simulink model "openloop_motor_with_sources_2020a"  (R2022a)
settings: Solver=VariableStepAuto  StartTime=0.0  StopTime=2  MaxStep=1e-6  MinStep=1e-12  RelTol=1e-3
values from neighbouring files (symbols this model uses):
  J = 0.02    [parameter.mat]
  Llr = 0.01033    [parameter.mat]
  Lls = 0.01033    [parameter.mat]
  Lm = 0.3197    [parameter.mat]
  Lr = 0.33003    [parameter.mat]
  Ls = 0.33003    [parameter.mat]
  np = 2    [parameter.mat]
  Rr = 2.178    [parameter.mat]
  Rs = 2.804    [parameter.mat]
  Tr = 0.15152892562    [parameter.mat]
undefined symbols (not defined in the file or in its folder): f, theta
libraries: spsACVoltageSourceLib x3, spsVoltageMeasurementLib x3, spsGroundLib x2, spsAsynchronousMachineSIUnitsLib x1, spspowerguiLib x1
settings Model: Creator=EVA  LastModifiedBy=EVA
settings SolverCC: AlgebraicLoopSolver=TrustRegion

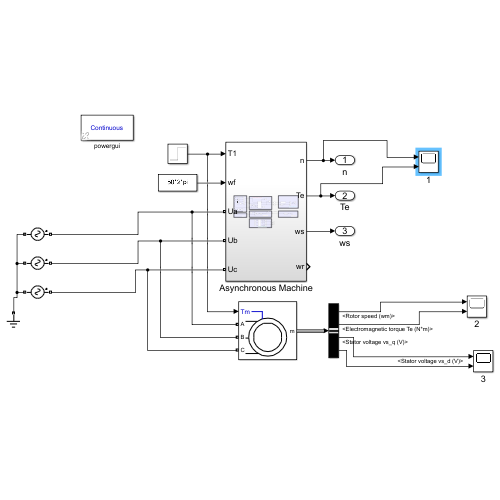
[thumbnail: Simulink's stored preview of the top-level diagram]
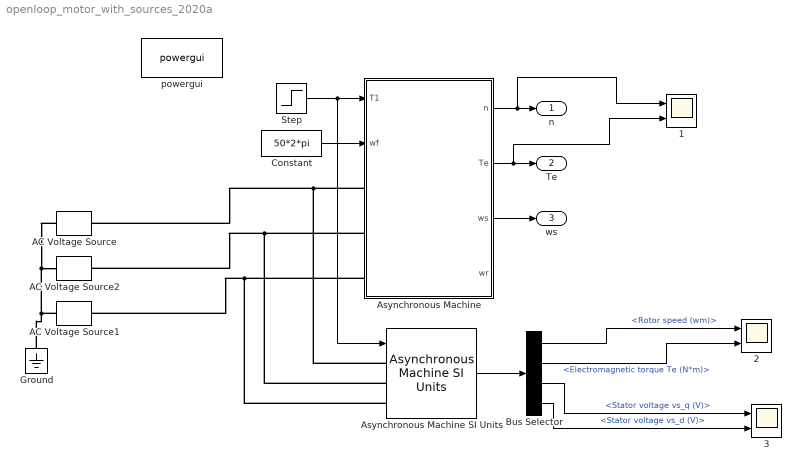
== system openloop_motor_with_sources_2020a ==
  1 : Scope  NumInputPorts=2
  2 : Scope  NumInputPorts=2
  3 : Scope  NumInputPorts=2
  AC Voltage Source : spsACVoltageSourceLib/AC Voltage Source  Amplitude=380  Phase=theta  Frequency=50  SampleTime=0  Measurements=None  BusType=swing  Pref=10e3  Qref=0  Qmin=-inf  Qmax=+inf
  AC Voltage Source1 : spsACVoltageSourceLib/AC Voltage Source  Amplitude=380  Phase=-240+theta  Frequency=50  SampleTime=0  Measurements=None  BusType=swing  Pref=10e3  Qref=0  Qmin=-inf  Qmax=+inf
  AC Voltage Source2 : spsACVoltageSourceLib/AC Voltage Source  Amplitude=380  Phase=-120+theta  Frequency=50  SampleTime=0  Measurements=None  BusType=swing  Pref=10e3  Qref=0  Qmin=-inf  Qmax=+inf
  Asynchronous Machine : Subsystem
  Asynchronous Machine SI Units : spsAsynchronousMachineSIUnitsLib/Asynchronous Machine SI Units  RotorType=Squirrel-cage  PresetModel=No  MechanicalLoad=Torque Tm  ShowDetailedParameters=on  ReferenceFrame=Rotor  Units=SI  MeasurementBus=off  NominalParameters=[1.845e+03 268 f]  VoltageRatio=1  Stator=[Rs Lls]  Rotor=[Rr Llr]  Cage1=[0.4155 0.002066]  Cage2=[0.4168 0.0003495]  Lm=Lm  Mechanical=[J 0.0 np]  PolePairs=2  InitialConditions=[1 0 0 0 0 0 0 0]  SimulateSaturation=off  Saturation=[14.03593122, 27.81365428, 53.79336849, 72.68890987, 97.98006896, 148.6815601, 215.7428561, 302.9841135, 428.7778367 ; 230, 322, 414, 460, 506, 552, 598, 644, 690]  LoadFlowParameters=1492000  TsPowergui=0  TsBlock=-1  IterativeModel=Trapezoidal non iterative  IterativeDiscreteModel=Trapezoidal non iterative  Pmec=0
  Bus Selector : BusSelector  OutputSignals=Mechanical.Rotor speed (wm),Mechanical.Electromagnetic torque Te (N*m),Stator measurements.Stator voltage vs_q (V),Stator measurements.Stator voltage vs_d (V)
  Constant : Constant  Value=50*2*pi
  Ground : spsGroundLib/Ground  LConnTagsString=a
  Step : Step  After=5  SampleTime=0
  powergui : spspowerguiLib/powergui  Priority=1  SimulationMode=Continuous  SampleTime=1e-7  frequency=60  Iterations=50  frequencyindice=50  Pbase=100e6  ErrMax=1e-4  UnitsV=kV  UnitsW=MW  buscounter=0  FunctionMessages=off  echomessages=off  EnableUseOfTLC=off  CurrentSourceSwitches=off  DisableSnubberDevices=off  DisableRonSwitches=off  DisableVfSwitches=off  DisplayEquations=off  AutomaticDiscreteSolvers=off  SolverType=Tustin/Backward Euler (TBE)  Interpol=off  ExternalGateDelay=off  methode=off  Ts=100  x0status=blocks  SPID=on  SwTol=0  HookPort=off  NonlinearTolerance=1e-4  nMaxIteration=100  ContinueOnMaxIteration=off  RestoreLinks=warning  ResistiveCurrentMeasurement=off  Frange=[0:2:500]  Ylog=off  Xlog=on  ShowGrid=off  save=off  variable=ZData  structure=0  ZoomFFT=off  StartTime=0.0  cycles=1  DisplayStyle=1  fundamental=60  FreqAxis=off  MaxFrequency=1000  frequencyindicesteady=1  RmsSteady=1  display=off
  n : Outport
  Te : Outport  Port=2
  ws : Outport  Port=3
  wires:
  Asynchronous Machine/1(n) -> 1/1, n/1
  Constant/1 -> Asynchronous Machine/2(wf)
  Asynchronous Machine/2(Te) -> 1/2, Te/1
  Step/1 -> Asynchronous Machine SI Units/1, Asynchronous Machine/1(T1)
  Asynchronous Machine/3(ws) -> ws/1
  Asynchronous Machine SI Units/1 -> Bus Selector/1
  Bus Selector/1 -> 2/1  "<Rotor speed (wm)>"
  Bus Selector/2 -> 2/2  "<Electromagnetic torque Te (N*m)>"
  Bus Selector/3 -> 3/1  "<Stator voltage vs_q (V)>"
  Bus Selector/4 -> 3/2  "<Stator voltage vs_d (V)>"
  connections:
  AC Voltage Source1/LConn1 -- Ground/LConn1 -- AC Voltage Source/LConn1 -- AC Voltage Source2/LConn1
  Asynchronous Machine/LConn1 -- Asynchronous Machine SI Units/LConn1 -- AC Voltage Source/RConn1
  Asynchronous Machine/LConn2 -- Asynchronous Machine SI Units/LConn2 -- AC Voltage Source2/RConn1
  Asynchronous Machine/LConn3 -- Asynchronous Machine SI Units/LConn3 -- AC Voltage Source1/RConn1

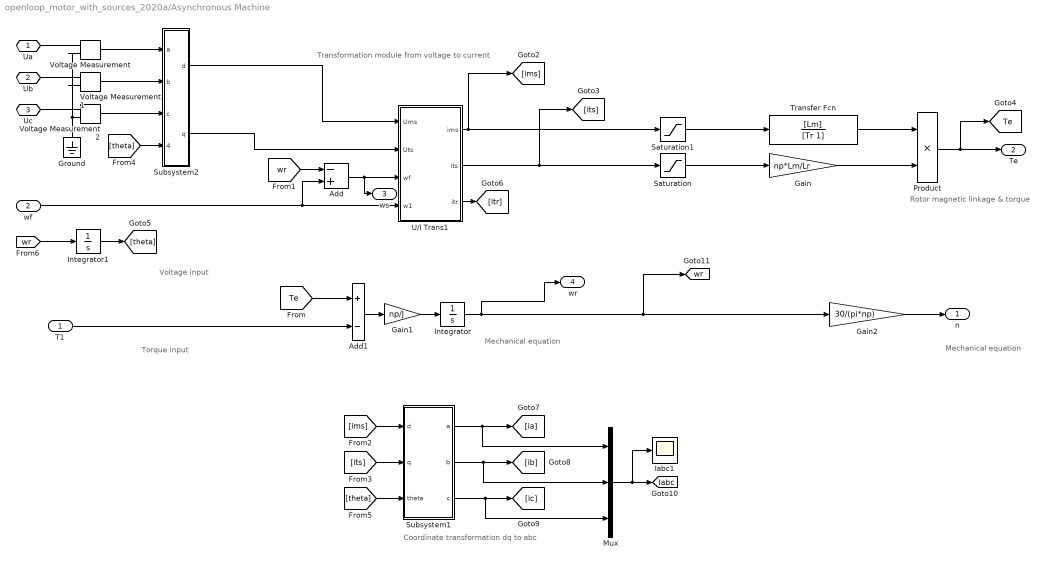
== system openloop_motor_with_sources_2020a/Asynchronous Machine ==
  note: Torque input
  note: Voltage input
  note: Rotor magnetic linkage & torque
  note: Transformation module from voltage to current
  note: Mechanical equation
  note: Coordinate transformation dq to abc
  note: Mechanical equation
  T1 : Inport
  wf : Inport  Port=2
  Add : Sum  Inputs=-+
  Add1 : Sum  Inputs=+-
  Gain : Gain  Gain=np*Lm/Lr
  Gain1 : Gain  Gain=np/J
  Gain2 : Gain  Gain=30/(pi*np)
  Ground : spsGroundLib/Ground  LConnTagsString=a
  Iabc1 : Scope
  Integrator : Integrator
  Integrator1 : Integrator
  Mux : Mux  Inputs=3
  Product : Product
  Saturation : Saturate  UpperLimit=50  LowerLimit=-50
  Saturation1 : Saturate  UpperLimit=50  LowerLimit=-50
  Subsystem1 : Subsystem
  Subsystem2 : Subsystem
  Transfer Fcn : TransferFcn  Numerator=[Lm]  Denominator=[Tr 1]
  U/I Trans1 : Subsystem
  Voltage Measurement : spsVoltageMeasurementLib/Voltage Measurement  PhasorSimulation=off  OutputType=Complex  PSBequivalent=0
  Voltage Measurement1 : spsVoltageMeasurementLib/Voltage Measurement  PhasorSimulation=off  OutputType=Complex  PSBequivalent=0
  Voltage Measurement2 : spsVoltageMeasurementLib/Voltage Measurement  PhasorSimulation=off  OutputType=Complex  PSBequivalent=0
  Ua : PMIOPort  Side=Left
  Ub : PMIOPort  Port=2  Side=Left
  Uc : PMIOPort  Port=3  Side=Left
  n : Outport
  Te : Outport  Port=2
  ws : Outport  Port=3
  wr : Outport  Port=4
  tag scope: Iabc=global, Te=global, wr=global
  wires:
  Subsystem1/3(c) -> Mux/3, [ic]
  wf/1 -> U/I Trans1/4(w1), Add/2
  Product/1 -> Te/1, [Te]
  U/I Trans1/2(its) -> Saturation/1, [its]
  Voltage Measurement2/1 -> Subsystem2/3(c)
  [theta] -> Subsystem2/4(theta)
  Gain2/1 -> n/1
  Add/1 -> ws/1, U/I Trans1/3(wf)
  U/I Trans1/1(ims) -> Saturation1/1, [ims]
  Add1/1 -> Gain1/1
  [theta] -> Subsystem1/3(theta)
  Voltage Measurement1/1 -> Subsystem2/2(b)
  Subsystem2/1(d) -> U/I Trans1/1(Ums)
  [its] -> Subsystem1/2(q)
  Voltage Measurement/1 -> Subsystem2/1(a)
  T1/1 -> Add1/2
  U/I Trans1/3(itr) -> [itr]
  [ims] -> Subsystem1/1(d)
  Integrator1/1 -> [theta]
  Integrator/1 -> [wr], Gain2/1, wr/1
  [wr] -> Add/1
  Gain1/1 -> Integrator/1
  Gain/1 -> Product/2
  Subsystem2/2(q) -> U/I Trans1/2(Uts)
  [Te] -> Add1/1
  Subsystem1/1(a) -> Mux/1, [ia]
  Subsystem1/2(b) -> Mux/2, [ib]
  Transfer Fcn/1 -> Product/1
  Mux/1 -> Iabc1/1, [Iabc]
  Saturation/1 -> Gain/1
  Saturation1/1 -> Transfer Fcn/1
  [wr] -> Integrator1/1
  connections:
  Ground/LConn1 -- Voltage Measurement1/LConn2 -- Voltage Measurement/LConn2 -- Voltage Measurement2/LConn2
  Uc/RConn1 -- Voltage Measurement2/LConn1
  Ub/RConn1 -- Voltage Measurement1/LConn1
  Ua/RConn1 -- Voltage Measurement/LConn1

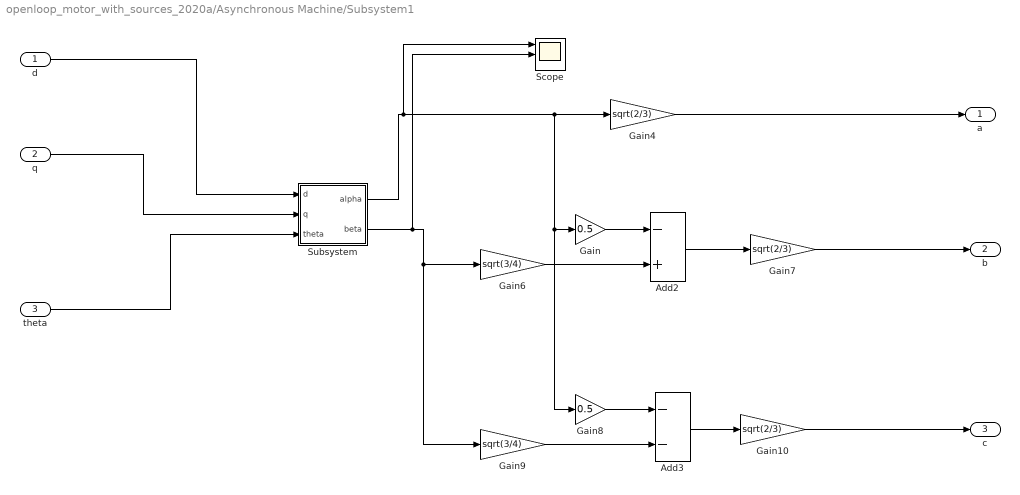
== system openloop_motor_with_sources_2020a/Asynchronous Machine/Subsystem1 ==
  d : Inport
  q : Inport  Port=2
  theta : Inport  Port=3
  Add2 : Sum  Inputs=-+
  Add3 : Sum  Inputs=--
  Gain : Gain  Gain=0.5
  Gain10 : Gain  Gain=sqrt(2/3)
  Gain4 : Gain  Gain=sqrt(2/3)
  Gain6 : Gain  Gain=sqrt(3/4)
  Gain7 : Gain  Gain=sqrt(2/3)
  Gain8 : Gain  Gain=0.5
  Gain9 : Gain  Gain=sqrt(3/4)
  Scope : Scope  NumInputPorts=3
  Subsystem : Subsystem
  a : Outport
  b : Outport  Port=2
  c : Outport  Port=3
  wires:
  Gain10/1 -> c/1
  Gain4/1 -> a/1
  Subsystem/2(beta) -> Scope/2, Gain9/1, Gain6/1
  q/1 -> Subsystem/2(q)
  theta/1 -> Subsystem/3(theta)
  d/1 -> Subsystem/1(d)
  Gain6/1 -> Add2/2
  Subsystem/1(alpha) -> Scope/1, Gain8/1, Gain/1, Gain4/1
  Add2/1 -> Gain7/1
  Gain9/1 -> Add3/2
  Gain7/1 -> b/1
  Add3/1 -> Gain10/1
  Gain/1 -> Add2/1
  Gain8/1 -> Add3/1

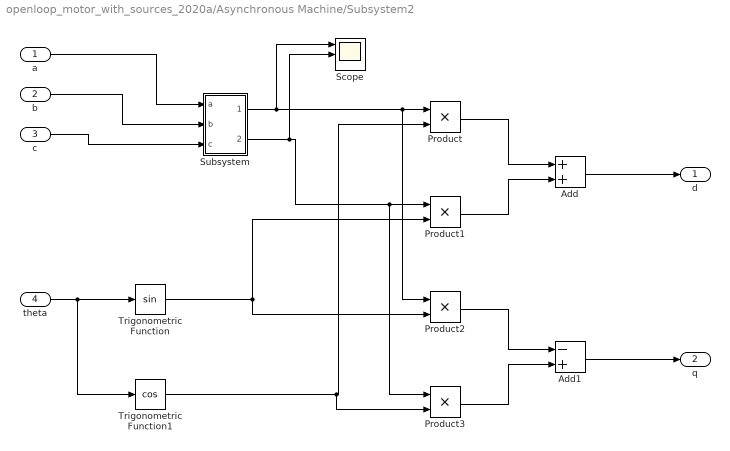
== system openloop_motor_with_sources_2020a/Asynchronous Machine/Subsystem2 ==
  a : Inport
  b : Inport  Port=2
  c : Inport  Port=3
  theta : Inport  Port=4
  Add : Sum
  Add1 : Sum  Inputs=-+
  Product{,1..3} (4 alike) : Product
  Scope : Scope  NumInputPorts=3
  Subsystem : Subsystem
  Trigonometric Function : Trigonometry
  Trigonometric Function1 : Trigonometry  Operator=cos
  d : Outport
  q : Outport  Port=2
  wires:
  Trigonometric Function1/1 -> Product3/2, Product/2
  Trigonometric Function/1 -> Product2/2, Product1/2
  Product/1 -> Add/1
  c/1 -> Subsystem/3(c)
  Subsystem/2(beta) -> Scope/2, Product3/1, Product1/1
  a/1 -> Subsystem/1(a)
  Product1/1 -> Add/2
  b/1 -> Subsystem/2(b)
  Subsystem/1(alpha) -> Scope/1, Product2/1, Product/1
  Product3/1 -> Add1/2
  theta/1 -> Trigonometric Function1/1, Trigonometric Function/1
  Product2/1 -> Add1/1
  Add1/1 -> q/1
  Add/1 -> d/1

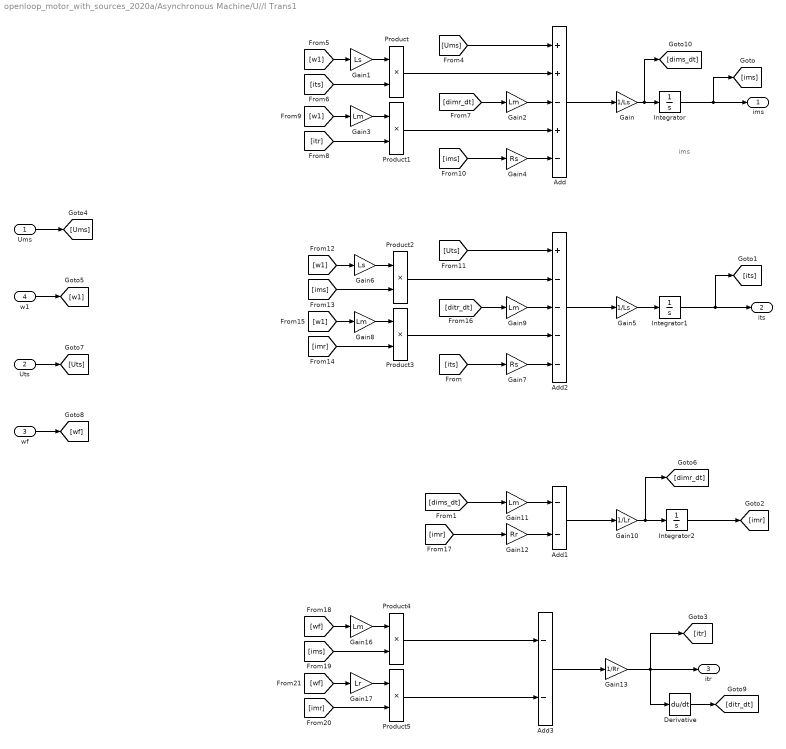
== system openloop_motor_with_sources_2020a/Asynchronous Machine/U//I Trans1 ==
  note: ims
  Ums : Inport
  Uts : Inport  Port=2
  wf : Inport  Port=3
  w1 : Inport  Port=4
  Add : Sum  Inputs=++-+-
  Add1 : Sum  Inputs=--
  Add2 : Sum  Inputs=+----
  Add3 : Sum  Inputs=--
  Derivative : Derivative
  Gain : Gain  Gain=1/Ls
  Gain1 : Gain  Gain=Ls
  Gain10 : Gain  Gain=1/Lr
  Gain{2..3,8..9,11,16} (6 alike) : Gain  Gain=Lm
  Gain12 : Gain  Gain=Rr
  Gain13 : Gain  Gain=1/Rr
  Gain17 : Gain  Gain=Lr
  Gain4 : Gain  Gain=Rs
  Gain5 : Gain  Gain=1/Ls
  Gain6 : Gain  Gain=Ls
  Gain7 : Gain  Gain=Rs
  Integrator : Integrator
  Integrator1 : Integrator
  Integrator2 : Integrator
  Product{,1..5} (6 alike) : Product
  ims : Outport
  its : Outport  Port=2
  itr : Outport  Port=3
  wires:
  Gain6/1 -> Product2/1
  [dimr_dt] -> Gain2/1
  Gain/1 -> Integrator/1, [dims_dt]
  Product2/1 -> Add2/2
  Gain8/1 -> Product3/1
  Add/1 -> Gain/1
  w1/1 -> [w1]
  Gain10/1 -> [dimr_dt], Integrator2/1
  wf/1 -> [wf]
  Integrator/1 -> ims/1, [ims]
  [dims_dt] -> Gain11/1
  [ims] -> Product4/2
  Gain9/1 -> Add2/3
  [imr] -> Product3/2
  [itr] -> Product1/2
  Gain2/1 -> Add/3
  [w1] -> Gain8/1
  [wf] -> Gain16/1
  Product3/1 -> Add2/4
  Integrator1/1 -> its/1, [its]
  Gain13/1 -> itr/1, Derivative/1, [itr]
  [w1] -> Gain3/1
  Gain16/1 -> Product4/1
  Gain5/1 -> Integrator1/1
  [Ums] -> Add/1
  [Uts] -> Add2/1
  Integrator2/1 -> [imr]
  Product4/1 -> Add3/1
  [its] -> Gain7/1
  Product1/1 -> Add/4
  Ums/1 -> [Ums]
  [imr] -> Product5/2
  Gain1/1 -> Product/1
  [ims] -> Product2/2
  [w1] -> Gain6/1
  [wf] -> Gain17/1
  [imr] -> Gain12/1
  Product/1 -> Add/2
  Gain11/1 -> Add1/1
  Uts/1 -> [Uts]
  Gain4/1 -> Add/5
  [ims] -> Gain4/1
  Gain7/1 -> Add2/5
  Add1/1 -> Gain10/1
  [its] -> Product/2
  Derivative/1 -> [ditr_dt]
  Add2/1 -> Gain5/1
  Product5/1 -> Add3/2
  Gain17/1 -> Product5/1
  Gain3/1 -> Product1/1
  [ditr_dt] -> Gain9/1
  [w1] -> Gain1/1
  Gain12/1 -> Add1/2
  Add3/1 -> Gain13/1

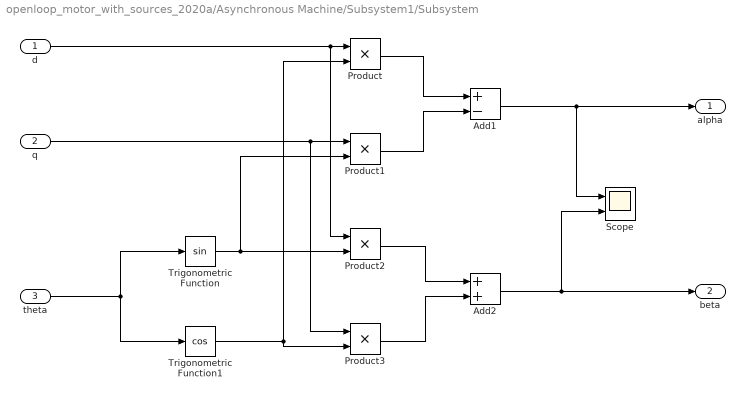
== system openloop_motor_with_sources_2020a/Asynchronous Machine/Subsystem1/Subsystem ==
  d : Inport
  q : Inport  Port=2
  theta : Inport  Port=3
  Add1 : Sum  Inputs=+-
  Add2 : Sum
  Product{,1..3} (4 alike) : Product
  Scope : Scope  NumInputPorts=2
  Trigonometric Function : Trigonometry
  Trigonometric Function1 : Trigonometry  Operator=cos
  alpha : Outport
  beta : Outport  Port=2
  wires:
  Product/1 -> Add1/1
  Add1/1 -> Scope/1, alpha/1
  q/1 -> Product3/1, Product1/1
  Product2/1 -> Add2/1
  Product1/1 -> Add1/2
  Trigonometric Function/1 -> Product2/2, Product1/2
  Product3/1 -> Add2/2
  Add2/1 -> Scope/2, beta/1
  d/1 -> Product2/1, Product/1
  theta/1 -> Trigonometric Function/1, Trigonometric Function1/1
  Trigonometric Function1/1 -> Product/2, Product3/2

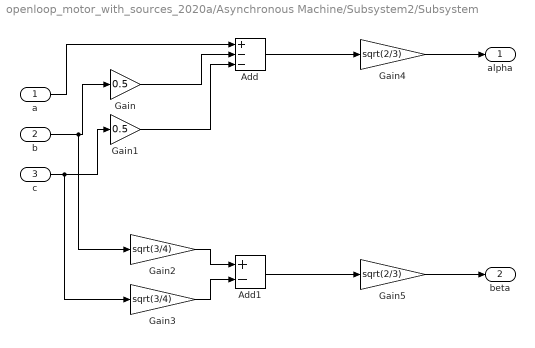
== system openloop_motor_with_sources_2020a/Asynchronous Machine/Subsystem2/Subsystem ==
  a : Inport
  b : Inport  Port=2
  c : Inport  Port=3
  Add : Sum  Inputs=+--
  Add1 : Sum  Inputs=+-
  Gain : Gain  Gain=0.5
  Gain1 : Gain  Gain=0.5
  Gain2 : Gain  Gain=sqrt(3/4)
  Gain3 : Gain  Gain=sqrt(3/4)
  Gain4 : Gain  Gain=sqrt(2/3)
  Gain5 : Gain  Gain=sqrt(2/3)
  alpha : Outport
  beta : Outport  Port=2
  wires:
  Add/1 -> Gain4/1
  b/1 -> Gain2/1, Gain/1
  Gain2/1 -> Add1/1
  Gain4/1 -> alpha/1
  Add1/1 -> Gain5/1
  c/1 -> Gain3/1, Gain1/1
  Gain/1 -> Add/2
  Gain3/1 -> Add1/2
  Gain5/1 -> beta/1
  a/1 -> Add/1
  Gain1/1 -> Add/3
